simulink model "stm32f4_exti_customcode_demo"  (Simulink 7.3)
settings: Solver=FixedStepDiscrete  SolverMode=SingleTasking  StartTime=0.0  StopTime=10.0  RelTol=1e-3
PreLoadFcn:
  | waijung.modelPreload; % Required for working with Waijung Blockset. Do not remove.
undefined symbols (not defined in the file): Button1, Drive1, enable_exti_customcode, HSEOSC, Link, LQFP176, Sensor1, Sensor2, ST, STM32F417IG, Switch1, Switch2
libraries: waijung_customcode x3, simulink x2, stm32f4_io_lib x1, stm32f4_device_config_lib x1
CloseFcn:
  | waijung.modelClose; % Required for working with Waijung Blockset. Do not remove.
settings Model: Creator=Krisada  LastModifiedBy=Krisada
settings OptimizationCC: OptimizeModelRefInitCode=on  LifeSpan=1
settings HardwareCC: ProdEndianess=LittleEndian  ProdHWDeviceType=ARM Compatible->Cortex - M4  TargetEndianess=LittleEndian  TargetHWDeviceType=ARM Compatible->Cortex - M4
settings RTWCC: SystemTargetFile=stm32f4.tlc  GenerateMakefile=off  TemplateMakefile=ert_default_tmf  Description=STM32F4 Target  ProcessScript=stm32f4_make_rtw_hook
settings CodeAppCC: IgnoreCustomStorageClasses=off
settings STFCustomTargetCC: ModelReferenceCompliant=off  CombineOutputUpdateFcns=on  ERTCustomFileBanners=on  SupportContinuousTime=off  SupportNonInlinedSFcns=off  SystemTargetFile=stm32f4.tlc
settings ERTTargetCC: MultiwordLength=2048  ModelReferenceCompliant=off  ParMdlRefBuildCompliant=off  CompOptLevelCompliant=off  ERTFirstTimeCompliant=off  ModelStepFunctionPrototypeControlCompliant=off  CPPClassGenCompliant=off  ExtModeMexFile=noextcomm  InlinedParameterPlacement=NonHierarchical  ERTSrcFileBannerTemplate=stm32f4_code_template.cgt  ERTHdrFileBannerTemplate=stm32f4_code_template.cgt  ERTDataSrcFileTemplate=stm32f4_code_template.cgt  ERTDataHdrFileTemplate=stm32f4_code_template.cgt  ERTCustomFileTemplate=stm32f4_file_process.tlc

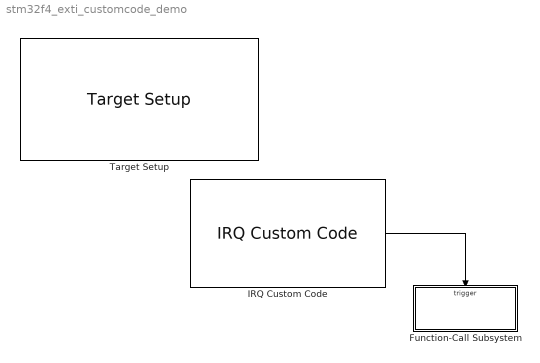
== system stm32f4_exti_customcode_demo ==
  Function-Call Subsystem : Subsystem  TreatAsAtomicUnit=on
  IRQ Custom Code : waijung_customcode/IRQ Custom Code  inputporttype=""  cinputportlabelstr="[\"\"]"  inputportcount=0  inputporttypeid=[-1]  outputporttype=uint32  coutputportlabel=IRQ  coutputportlabelstr="[\"IRQ\"]"  outputportcount=1  outputporttypeid=[7]  incpath={stm32f4incpath, fullfile(pwd,'exti_customcode')}  srcpath={stm32f4srcpath, fullfile(pwd,'exti_customcode')}  incfiles={'stm32f4xx_gpio.h';'stm32f4xx_exti.h'; 'exti_customcode.h'}  srcfiles={'stm32f4xx_gpio.c','stm32f4xx_exti.c', 'exti_customcode.c'}  initialfuncallstr=/* Write block start-up code here */  enablefuncallstr=enable_exti_customcode();  outputfuncallstr=void EXTI0_IRQHandler (void)  disablefuncallstr=/* disable_exti_customcode(); */  sampletime=inf  sampletimestr=Inf  blockid=IRQCustomCode  enablecustomportlabel=on  incfilestrarray="[\"stm32f4xx_gpio.h\",\"stm32f4xx_exti.h\",\"exti_customcode.h\"]"
  Target Setup : stm32f4_device_config_lib/Target Setup  Priority=100  compiler=GNU ARM  previous_compiler=GNU ARM  mcu=STM32F417IG (LQFP176)  mcustr=STM32F417IG  clockconfig=HSEOSC-8MHz  system_stm32f4xx_c_path=F:\trunk\targets\stm32f4_target\stm32f4\utils\system_stm32f4xx_default\STM32F40_41xxx\hseosc8mhz  showmemoryconfiguration=off  stacksize=0x2000  heapsize=0x2000  enableautocompiledownload=on  fullchiperase=off  programmerinterface=ST-Link  editctrlstr=on  compilercontrolstr=$(patsubst %, -I%, .) -mcpu=cortex-m4 -mthumb -mthumb-interwork -mfloat-abi=hard -mfpu=fpv4-sp-d16 -ffast-math -Wall -Wextra -Ofast  assemblercontrolstr=$(patsubst %, -I%, .) -mcpu=cortex-m4 -mthumb -mthumb-interwork -mfloat-abi=hard -mfpu=fpv4-sp-d16 -ffast-math -Wall -Wextra -Ofast -Wa,-amhls=$(<:.s=.lst) -D__STACK_SIZE=$(STACK_SIZE) -D__HEAP_SIZE=$(HEAP_SIZE)  linkercontrolstr=-T$(LD_SCRIPT) -g -Wl,-Map=$(MAP),--cref,--no-warn-mismatch -mcpu=cortex-m4 -mthumb -mthumb-interwork -mfloat-abi=hard -mfpu=fpv4-sp-d16 -specs=nosys.specs  runafterdownload=on  execprofile=None  profileruart=3  profilerbaud=500000  profilertxpin=D8  profilerinitstr=0.01,168000000,1680000,500000,0  manualsetsampletime=off  sampletime=0.01  blockid=TargetSetup  systickreloadvalue=1680000  hseval=8000000  lastprofileruart=3  hclk=168000000  flashorigin=0x8000000  flashlength=1024k  ramorigin=0x20000000  ramlength=128k  useextram=off
  wires:
  IRQ Custom Code/1 -> Function-Call Subsystem/Trigger

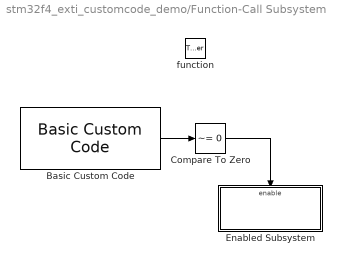
== system stm32f4_exti_customcode_demo/Function-Call Subsystem ==
  function : TriggerPort  TriggerType=function-call
  Basic Custom Code : waijung_customcode/Basic Custom Code  inputporttype=""  cinputportlabel=Sensor1,Sensor2,Switch1,Switch2  cinputportlabelstr="[\"Sensor1\",\"Sensor2\",\"Switch1\",\"Switch2\"]"  inputportcount=0  inputporttypeid=[-1]  outputporttype=uint32  coutputportlabel=IT_Status  coutputportlabelstr="[\"IT_Status\"]"  outputportcount=1  outputporttypeid=[7]  incpath={}  srcpath={}  incfiles={}  srcfiles={}  outputfuncallstr={ uint32_t reg_val; reg_val = (uint32_t) EXTI_GetITStatus(EXTI_Line0); *out1 = reg_val;}  sampletime=inf  sampletimestr=-1  blockid=FunctionCallSubsystemBasicCustomCode  enablecustomportlabel=on  incfilestrarray=[]  inputportdiminfo=[]  outputportdiminfo="[1  1  1  7]"
  Compare To Zero : simulink/Logic and Bit Operations/Compare To Zero  SystemSampleTime=-1  relop=~=  LogicOutDataTypeMode=uint8  ZeroCross=off
  Enabled Subsystem : Subsystem  TreatAsAtomicUnit=on
  wires:
  Basic Custom Code/1 -> Compare To Zero/1
  Compare To Zero/1 -> Enabled Subsystem/Enable

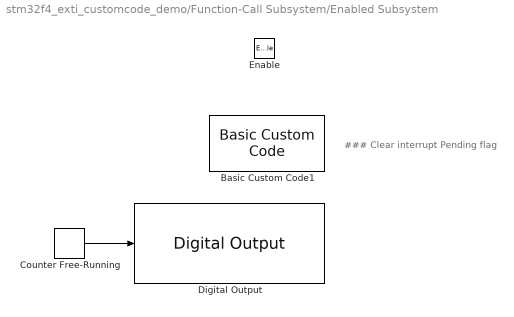
== system stm32f4_exti_customcode_demo/Function-Call Subsystem/Enabled Subsystem ==
  note: ### Clear interrupt Pending flag
  Enable : EnablePort
  Basic Custom Code1 : waijung_customcode/Basic Custom Code  inputporttype=""  cinputportlabel=Sensor1,Sensor2,Switch1,Switch2  cinputportlabelstr="[\"Sensor1\",\"Sensor2\",\"Switch1\",\"Switch2\"]"  inputportcount=0  inputporttypeid=[-1]  outputporttype=""  coutputportlabel=Drive1,Button1  coutputportlabelstr="[\"Drive1\",\"Button1\"]"  outputportcount=0  outputporttypeid=[-1]  incpath={}  srcpath={}  incfiles={}  srcfiles={}  outputfuncallstr={ EXTI_ClearITPendingBit(EXTI_Line0); }  sampletime=inf  sampletimestr=-1  blockid=FunctionCallSubsystemEnabledSubsystemBasicCustomCode1  enablecustomportlabel=on  incfilestrarray=[]  inputportdiminfo=[]  outputportdiminfo=[]
  Counter Free-Running : simulink/Sources/Counter Free-Running  SystemSampleTime=-1  NumBits=16  tsamp=-1
  Digital Output : stm32f4_io_lib/Digital Output  use_bitband=on  port=D  speed=100  porttype=Push Pull  porttypestr=PP  use_pin0=off  use_pin1=off  use_pin2=off  use_pin3=off  use_pin4=off  use_pin5=off  use_pin6=off  use_pin7=off  use_pin8=off  use_pin9=off  use_pin10=off  use_pin11=off  use_pin12=off  use_pin13=off  use_pin14=off  use_pin15=on  pinstr=GPIO_Pin_15  usedpinarray="[0  0  0  0  0  0  0  0  0  0  0  0  0  0  0  1]"  bitbandingstr="#define FunctionCallSubsystemEnabledSubsystemDigitalOutput_D15 Peripheral_BB(GPIOD->ODR, 15)  /* Output pin */"  sampletime=-1  sampletimestr=-1  blockid=FunctionCallSubsystemEnabledSubsystemDigitalOutput  enablecustomportlabel=off  globalinit=off  cinputportlabel=In1, In2  coutputportlabel=0
  wires:
  Counter Free-Running/1 -> Digital Output/1
